simulink model "haleytut1_3"  (R2023b)
settings: Solver=FixedStepAuto  StartTime=0.0  StopTime=10  FixedStep=1e-3  RelTol=1e-3  EnableMultiTasking=on
libraries: frdmk64flib x1
settings Model: ExtModeTrigDuration=5  Creator=haley  LastModifiedBy=bardiased
settings OptimizationCC: EnhancedBackFolding=on  PassReuseOutputArgsAs=Individual arguments  ZeroExternalMemoryAtStartup=off  ZeroInternalMemoryAtStartup=off  MaxStackSize=64  OptimizeBlockOrder=speed  DifferentSizesBufferReuse=on  OptimizationCustomize=off  EfficientTunableParamExpr=on
settings DebuggingCC: ParameterTunabilityLossMsg=error
settings HardwareCC: ProdBitPerPointer=32  ProdBitPerSizeT=32  ProdBitPerPtrDiffT=32  ProdLargestAtomicInteger=Long  ProdLargestAtomicFloat=Double  ProdWordSize=32  ProdHWDeviceType=ARM Compatible->ARM Cortex
settings SFSimCC: MATLABDynamicMemAlloc=off
settings RTWCC: Description=Embedded Coder  SystemTargetFile=ert.tlc  HardwareBoard=NXP FRDM-K64F  TLCOptions="-aInlineSetEventsForThisBaseRateFcn=TLC_FALSE -aSuppressMultiTaskScheduler=TLC_FALSE  -aRateBasedStepFcn=0"  TemplateMakefile=ert_default_tmf  Toolchain=GNU Tools for ARM Embedded Processors
settings CodeAppCC: ForceParamTrailComments=on  IgnoreCustomStorageClasses=off  OperatorAnnotations=on  SimulinkDataObjDesc=on  SFDataObjDesc=on  InsertBlockDesc=on
settings ERTTargetCC: ExtModeTransport=4  ExtModeMexFile=sendToCommService

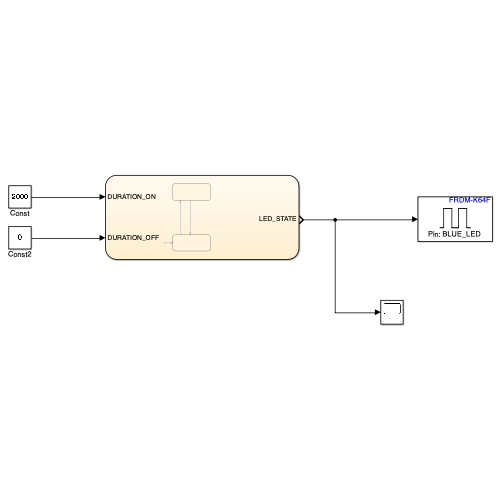
[thumbnail: Simulink's stored preview of the top-level diagram]
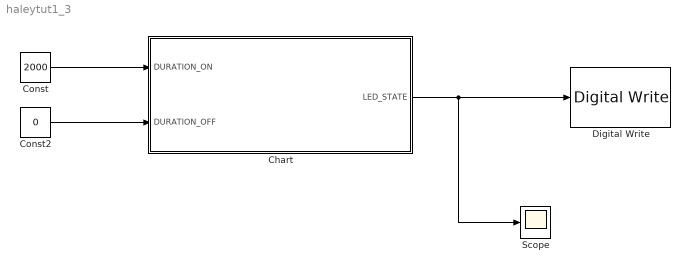
== system haleytut1_3 ==
  Chart : Stateflow chart  TreatAsAtomicUnit=on
  Const : Constant  Value=2000  OutDataTypeStr=int16
  Const2 : Constant  Value=0  OutDataTypeStr=int16
  Digital Write : frdmk64flib/Digital Write  Whichpin=BLUE_LED
  Scope : Scope
  wires:
  Chart/1(LED_STATE) -> Scope/1, Digital Write/1
  Const/1 -> Chart/1(DURATION_ON)
  Const2/1 -> Chart/2(DURATION_OFF)

== stateflow chart haleytut1_3/Chart ==
  state LED_ON
    entry:
    LED_STATE = true;
  state LED_OFF
    entry:
    LED_STATE = false;
  LED_OFF -> LED_ON : [after(DURATION_ON, msec)
      | ]
  LED_ON -> LED_OFF : [after(DURATION_OFF, msec)]
  (default) -> LED_OFF
  data: DURATION_ON input int16; DURATION_OFF input int16; LED_STATE output boolean
